simulink model "gSSVEP_gUSBamp_8ch"  (Simulink 8.6)
settings: Solver=FixedStepDiscrete  StartTime=0.0  StopTime=260  FixedStep=1/256  RelTol=1e-3
libraries: dspstat3 x2, Tools x1, dspbuff3 x1, gRTanalyze x1, simulink x1, gSTIMboxlib x1
Description:
  | g.USBamp based SSVEP based BCI
  | 
  | Copyright g.tec medical engineering GmbH
settings Model: Creator=g.tec medical engineering GmbH  ModifiedByFormat=g.tec  LastModifiedBy=g.tec
settings DebuggingCC: FcnCallInpInsideContextMsg=UseLocalSettings

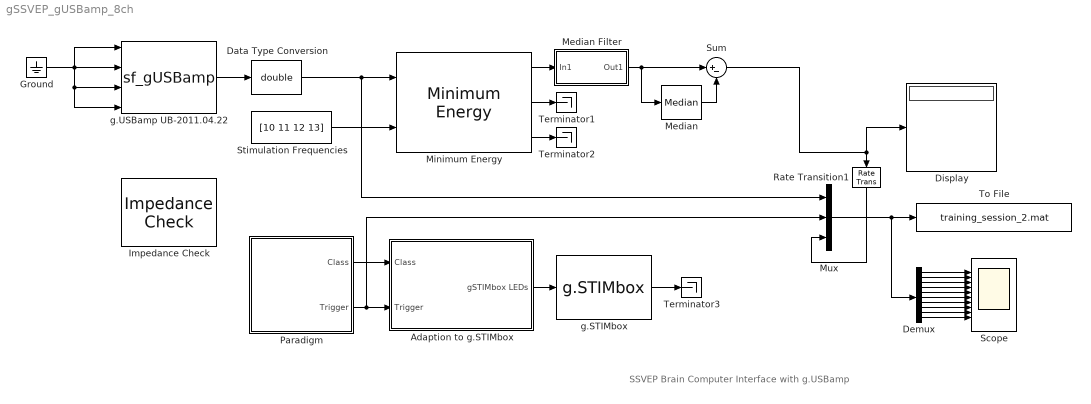
== system gSSVEP_gUSBamp_8ch ==
  note: SSVEP Brain Computer Interface with g.USBamp
  Adaption to g.STIMbox : Subsystem
      settings: MinAlgLoopOccurrences=on
  Data Type Conversion : DataTypeConversion  OutDataTypeStr=double
  Demux : Demux  Outputs=10
  Display : Display
  Ground : Ground
  Impedance Check : Tools/Impedance Check
  Median : dspstat3/Median  sortAlg=Quick sort  directionMode=Entire input  dimension=1  outputDataTypeStr=Inherit: Same as accumulator  outputLastDataTypeStr=Inherit: Same as accumulator  outputMin=[]  outputMax=[]  accumDataTypeStr=Inherit: Same as product output  accumLastDataTypeStr=Inherit: Same as product output  roundingMode=Floor  overflowMode=off
      settings: allowOverrides=off
  Median Filter : Subsystem  mask(Moving Median Filter){buflen=10}
      mask prompts: buflen "Filter Length"
      mask help:
      | Smoothes the input channels over time by computing the median value for
      | the specified number of samples.
      mask init:
      | blockhandle = get_param(gcb,'Handle');
      | sysname = get(blockhandle,'Path');
      | syspath = [ sysname '/' ];
      | name = [ syspath get(blockhandle,'Name') ];
      | path = [ name '/' ];
      | if buflen < 3
      |   buflen = 10;
      |   set_param(name,'buflen',num2str(buflen));
      | end
      | set_param([ path 'Collect'],'siz',num2str(buflen));
      | try
      |   set_param([ path 'Collect'],'TreatMby1Signals','M channels (this choice will be removed - see release notes)');
      | catch
      | end
      mask Help:
      | Smoothes the input channels over time by computing the median value for
      | the specified number of samples.
      | 
      | Filter Length ... The length of the smoothing window in samples. (Default 10)
  Minimum Energy : gRTanalyze/Minimum Energy  bufflen=768  reprate=0.20  numharmonics=1  modelorder=7
  Mux : Mux  Inputs=3
  Paradigm : Subsystem  mask{classinfo=classinfo_20tr.m, mode=Paradigm with feedback, trialperiod=10.5, activepart=70, initialoffset=10}
      mask prompts: classinfo "Class Info File"; trialperiod "Trial Period [s] (>= 8s)"; activepart "Active Part [%]"; initialoffset "Initial Offset [s] (>= 10s)"
      mask init:
      | blockhandle = get_param(gcb,'Handle');
      | sysname = get(blockhandle,'Path');
      | syspath = [ sysname '/' ];
      | name = [ syspath get(blockhandle,'Name') ];
      | path = [ name '/' ];
      | rootsys = bdroot(name);
      | 
      | if ~strcmp(get_param(rootsys, 'SolverType'),'Fixed-step')
      |         set_param(rootsys, 'SolverType','Fixed-step');
      | end
      |         
      | stepsize = get_param(rootsys,'FixedStep');
      | if strcmp(stepsize,'auto')
      |     error('Currently not known how to determine FixedStep size during initialization')
      | end
      | 
      | if mode==3    %Free Running
      |     paradigmDrivePattern = [ 0 , -1 ];
      |     
      | else   %Training paradigm or Paradigm with feedback
      |     try 
      |       ci = load(classinfo);
      |       cioffval = min(ci',[],1);
      |       [ cival ci ] = max(ci',[],1);
      |      % ci(end +1) = 0;
      |     catch
      |       fprintf(2,'File %s required check paths and session settings\n', classinfo);
      |       error('File %s required check paths and session settings', classinfo);
      |     end
      |  %   set_param([ path 'SetTrigger' ],'Value','1');
      |     
      |     if trialperiod < 8   %trialperiod should not be higher than 5s (could be removed if necessary)
      |       trialperiod = 8;
      |       set_param(name,'trialperiod','5');
      |     end
      |     if activepart > 95   %activepart should be lower than 95% (could be removed if necessary)
      |       activepart = 95;
      |       set_param(name,'activepart','95');
      |     end
      |     if initialoffset < 10   %initaloffset should be >= 0s
      |       initialoffset = 10;
      |       set_param(name,'initialoffset','0');
      |     end
      |     
      |     hightime = activepart / 100 * trialperiod;
      | 
      |     stepsize_int = str2num(stepsize);
      |     hightime = round(hightime / stepsize_int);
      |     trialperiod = round(trialperiod / stepsize_int);
      |     if hightime < 2 / stepsize_int    %hightime should not be lower than 2s (could be removed if necessary)
      |         hightime = 2 / stepsize_int;
      |     end
      |         
      |     offset_samp = round(initialoffset / stepsize_int);
      |         
      |     %activepart = hightime;
      |     array = zeros(1,trialperiod*size(ci,2)+offset_samp);
      |     for cnt=1:size(ci,2)
      |         put = ( cnt - 1) * trialperiod + 1 + offset_samp;
      |         put = put:(put+hightime-1);
      |         if cival(cnt) > 0
      |             array(1,put) = ci(cnt);
      |         elseif cioffval(cnt) < 0
      |             % do not flash at all, may be used to train for less
      |             % than 3 classes to be detected. Just generate the
      |             % trigger
      |             array(1,put) = inf;
      |         end
      |     end
      |     ci=array;
      |     ci = [ [0:( size(ci,2) - 1 )].*stepsize_int ; ci ];
      |     paradigmDrivePattern = ci';
      |             
      |     period = num2str(trialperiod,10);
      |     offset = num2str(initialoffset,10);
      | end
      | 
      | set_param([ path 'Class Info' ],'VariableName','paradigmDrivePattern');
      | set_param([ path 'Class Info' ],'SampleTime',stepsize);
      | 
      | clear blockhandle sysname syspath name path classinfo trialperiod activepart initialoffset
      settings: MinAlgLoopOccurrences=on
      mask TypeOptions mode: Training Paradigm | Paradigm with feedback | Free running
  Rate Transition1 : RateTransition
  Scope : Scope  NumInputPorts=10
  Stimulation Frequencies : Constant  Value=[10 11 12 13]  SampleTime=1/256
  Sum : Sum  Inputs=|+-
  Terminator1 : Terminator
  Terminator2 : Terminator
  Terminator3 : Terminator
  To File : ToFile  Filename=training_session_2.mat  MatrixName=y
  g.STIMbox : gSTIMboxlib/g.STIMbox  comport=3  sr=32  fl=1  ia=1  bm=0  fs=1  chmodes="[0  0  0  0  0  0  0  0  1  0  1  0  1  0  1  0]"  chfreqs="[1   1   1   1   1   1   1   1  10   1  11   1  12   1  13   1]"  chinv="[0  0  0  0  0  0  0  0  0  0  0  0  0  0]"
  g.USBamp UB-2011.04.22 : S-Function  FunctionName=sf_gUSBamp  Parameters=cfg,snr  SFunctionDeploymentMode=off  EnableBusSupport=off  mask{cfg=currentCFG_gSSVEP_gUSBamp_8ch_UB-2011.04.22.cfg, snr=UB-2011.04.22}
      mask prompts: cfg "Configuration"; snr "Serial"
      mask help: Enter configuration file and serial
      settings: OpenFcn=|
      | %gua_click
      | gua_block_cfg
      mask Display: image(imread('USB_symb.tif'))
  wires:
  Stimulation Frequencies/1 -> Minimum Energy/2
  Minimum Energy/1 -> Median Filter/1(In1)
  Median Filter/1(Out1) -> Sum/1, Median/1
  Minimum Energy/2 -> Terminator1/1
  Minimum Energy/3 -> Terminator2/1
  g.USBamp UB-2011.04.22/1 -> Data Type Conversion/1
  Data Type Conversion/1 -> Mux/1, Minimum Energy/1
  Paradigm/2(Trigger) -> Mux/2, Adaption to g.STIMbox/2(Trigger)
  Mux/1 -> To File/1, Demux/1
  Paradigm/1(Class) -> Adaption to g.STIMbox/1(Class)
  Rate Transition1/1 -> Mux/3
  Adaption to g.STIMbox/1(gSTIMbox LEDs) -> g.STIMbox/1
  g.STIMbox/1 -> Terminator3/1
  Demux/1 -> Scope/1
  Demux/2 -> Scope/2
  Demux/3 -> Scope/3
  Demux/4 -> Scope/4
  Demux/5 -> Scope/5
  Demux/6 -> Scope/6
  Demux/7 -> Scope/7
  Demux/8 -> Scope/8
  Demux/9 -> Scope/9
  Demux/10 -> Scope/10
  Median/1 -> Sum/2
  Ground/1 -> g.USBamp UB-2011.04.22/3, g.USBamp UB-2011.04.22/4, g.USBamp UB-2011.04.22/1, g.USBamp UB-2011.04.22/2
  Sum/1 -> Rate Transition1/1, Display/1

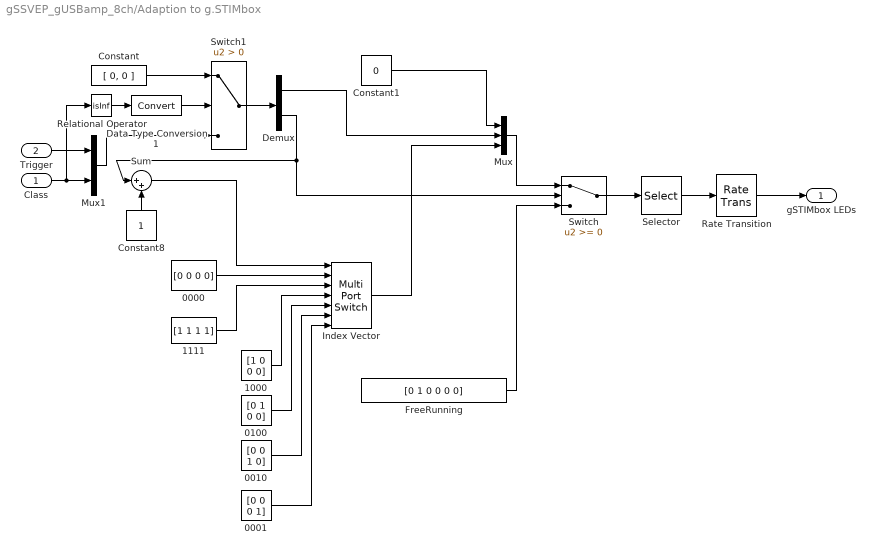
== system gSSVEP_gUSBamp_8ch/Adaption to g.STIMbox ==
  Class : Inport
  Trigger : Inport  Port=2
  0000 : Constant  Value=[0 0 0 0]  SampleTime=1/256
  0001 : Constant  Value=[0 0 0 1]  SampleTime=1/256
  0010 : Constant  Value=[0 0 1 0]  SampleTime=1/256
  0100 : Constant  Value=[0 1 0 0]  SampleTime=1/256
  1000 : Constant  Value=[1 0 0 0]  SampleTime=1/256
  1111 : Constant  Value=[1 1 1 1]  SampleTime=1/256
  Constant : Constant  Value=[ 0, 0 ]
  Constant1 : Constant  Value=0  SampleTime=1/256
  Constant8 : Constant  SampleTime=1/256
  Data Type Conversion1 : DataTypeConversion
  Demux : Demux  Outputs=2
  FreeRunning : Constant  Value=[0 1 0 0 0 0]  SampleTime=1/256
  Index Vector : MultiPortSwitch  DataPortOrder=Zero-based contiguous  Inputs=6  zeroidx=on
  Mux : Mux  Inputs=3
  Mux1 : Mux  Inputs=2
  Rate Transition : RateTransition
  Relational Operator : RelationalOperator  Operator=isInf  OutDataTypeStr=boolean
  Selector : Selector  InputPortWidth=6  IndexOptions=Index vector (dialog)  Indices=[ones(1,8) 2 3 2 4 2 5 2 6]  OutputSizes=1
  Sum : Sum  Inputs=|++
  Switch : Switch
  Switch1 : Switch  Criteria=u2 > Threshold
  gSTIMbox LEDs : Outport
  wires:
  Trigger/1 -> Mux1/1
  Constant1/1 -> Mux/1
  Index Vector/1 -> Mux/3
  Mux/1 -> Switch/1
  FreeRunning/1 -> Switch/3
  Switch/1 -> Selector/1
  Selector/1 -> Rate Transition/1
  Rate Transition/1 -> gSTIMbox LEDs/1
  Class/1 -> Relational Operator/1, Mux1/2
  Constant8/1 -> Sum/2
  Sum/1 -> Index Vector/1
  0000/1 -> Index Vector/2
  1111/1 -> Index Vector/3
  1000/1 -> Index Vector/4
  0100/1 -> Index Vector/5
  0010/1 -> Index Vector/6
  0001/1 -> Index Vector/7
  Relational Operator/1 -> Data Type Conversion1/1
  Data Type Conversion1/1 -> Switch1/2
  Constant/1 -> Switch1/1
  Switch1/1 -> Demux/1
  Mux1/1 -> Switch1/3
  Demux/1 -> Mux/2
  Demux/2 -> Sum/1, Switch/2

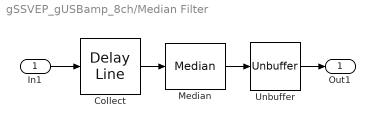
== system gSSVEP_gUSBamp_8ch/Median Filter ==
  In1 : Inport
  Collect : dspbuff3/Delay Line  siz=10  ic=0  directfeed=on  enable_output=off  hold_output=off  TreatMby1Signals=M channels (this choice will be removed - see release notes)  OutputFrames=on
  Median : dspstat3/Median  sortAlg=Quick sort  directionMode=Specified dimension  dimension=1  outputDataTypeStr=Inherit: Same as accumulator  outputLastDataTypeStr=Inherit: Same as accumulator  outputMin=[]  outputMax=[]  accumDataTypeStr=Inherit: Same as product output  accumLastDataTypeStr=Inherit: Same as product output  roundingMode=Floor  overflowMode=off
      settings: allowOverrides=off
  Unbuffer : Unbuffer
  Out1 : Outport
  wires:
  Unbuffer/1 -> Out1/1
  Median/1 -> Unbuffer/1
  Collect/1 -> Median/1
  In1/1 -> Collect/1

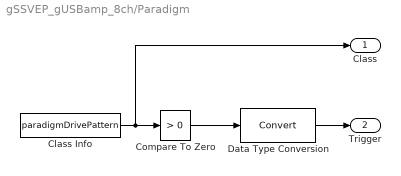
== system gSSVEP_gUSBamp_8ch/Paradigm ==
  Class Info : FromWorkspace  VariableName=paradigmDrivePattern  SampleTime=1/256  Interpolate=off  OutputAfterFinalValue=Holding final value
  Compare To Zero : simulink/Logic and Bit Operations/Compare To Zero  relop=>  OutDataTypeStr=uint8  ZeroCross=off
  Data Type Conversion : DataTypeConversion
  Class : Outport  InitialOutput=0
  Trigger : Outport  Port=2  InitialOutput=0
  wires:
  Class Info/1 -> Compare To Zero/1, Class/1
  Compare To Zero/1 -> Data Type Conversion/1
  Data Type Conversion/1 -> Trigger/1
